simulink model "RangingEstimatorV3Test200CM"  (R2020b)
settings: Solver=FixedStepDiscrete  StartTime=0.0  StopTime=1  FixedStep=0.000001  RelTol=1e-3  EnableMultiTasking=on
settings Model: Creator=拾夕  LastModifiedBy=拾夕
settings OptimizationCC: DefaultUnderspecifiedDataType=single  EnhancedBackFolding=on  PassReuseOutputArgsAs=Individual arguments  ZeroExternalMemoryAtStartup=off  ZeroInternalMemoryAtStartup=off  MaxStackSize=64  OptimizeBlockOrder=speed  DifferentSizesBufferReuse=on  OptimizationCustomize=off  EfficientTunableParamExpr=on
settings DebuggingCC: ParameterTunabilityLossMsg=error
settings HardwareCC: ProdBitPerInt=16  ProdBitPerPointer=16  ProdBitPerSizeT=16  ProdBitPerPtrDiffT=16  ProdLargestAtomicFloat=None  ProdWordSize=8  ProdHWDeviceType=Atmel->AVR
settings SFSimCC: MATLABDynamicMemAlloc=off
settings RTWCC: Description=Embedded Coder  SystemTargetFile=ert.tlc  HardwareBoard=Arduino Uno  TemplateMakefile=ert_default_tmf  GenerateReport=on  RetainRTWFile=on  Toolchain=Arduino AVR  BuildConfiguration=Faster Runs  LaunchReport=on  GenerateWebview=on  GenerateCodeMetricsReport=on
settings CodeAppCC: ForceParamTrailComments=on  IgnoreCustomStorageClasses=off  OperatorAnnotations=on  SimulinkDataObjDesc=on  SFDataObjDesc=on  InsertBlockDesc=on
settings ERTTargetCC: SupportContinuousTime=on  SupportVariableSizeSignals=on  ExtModeStaticAllocSize=250

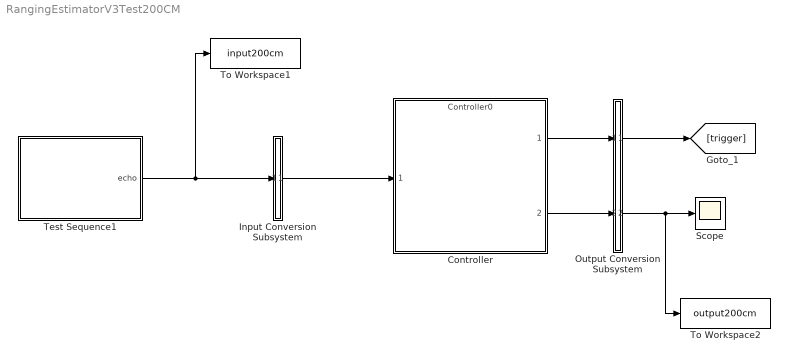
== system RangingEstimatorV3Test200CM ==
  Controller : ModelReference  ModelNameDialog=Controller0  SimulationMode=Normal  ModelReferenceVersion=1.24
  Input Conversion Subsystem : Subsystem  Tag=__SLT_ICS__  Description=|
      | Signal spec.
      | and routing
      settings: AttributesFormatString=%<Description>
  Output Conversion Subsystem : Subsystem  Tag=__SLT_OCS__  Description=|
      | Signal spec.
      | and routing
      settings: AttributesFormatString=%<Description>
  Scope : Scope
  Test Sequence1 : Test Sequence  TreatAsAtomicUnit=on
  To Workspace1 : ToWorkspace  VariableName=input200cm  SaveFormat=Timeseries  SampleTime=-1
  To Workspace2 : ToWorkspace  VariableName=output200cm  SaveFormat=Timeseries  SampleTime=-1
  wires:
  Output Conversion Subsystem/1(Outport_1) -> [trigger]
  Output Conversion Subsystem/2(Outport_2) -> To Workspace2/1, Scope/1
  Input Conversion Subsystem/1(Outport_1) -> Controller/1
  Controller/1 -> Output Conversion Subsystem/1(Inport_1)
  Controller/2 -> Output Conversion Subsystem/2(Inport_2)
  Test Sequence1/1(echo) -> To Workspace1/1, Input Conversion Subsystem/1(Inport_1)

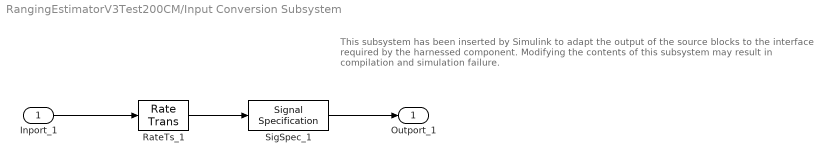
== system RangingEstimatorV3Test200CM/Input Conversion Subsystem ==
  note: This subsystem has been inserted by Simulink to adapt the output of the source blocks to the interface required by the harnessed component.
      |  Modifying the contents of this subsystem may result in compilation and simulation failure.
  Inport_1 : Inport
  RateTs_1 : RateTransition  OutPortSampleTime=1e-06
  SigSpec_1 : SignalSpecification  OutDataTypeStr=single  Dimensions=[1]  SampleTime=1e-06
  Outport_1 : Outport
  wires:
  SigSpec_1/1 -> Outport_1/1
  RateTs_1/1 -> SigSpec_1/1
  Inport_1/1 -> RateTs_1/1

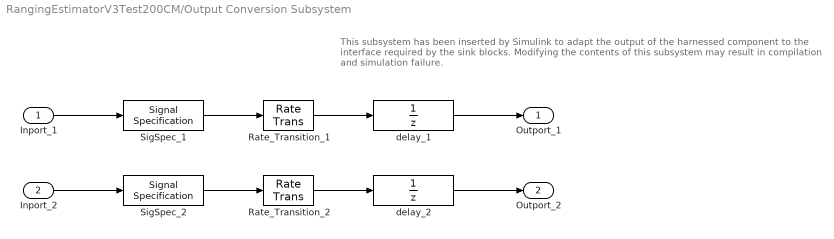
== system RangingEstimatorV3Test200CM/Output Conversion Subsystem ==
  note: This subsystem has been inserted by Simulink to adapt the output of the harnessed component to the interface required by the sink blocks.
      |  Modifying the contents of this subsystem may result in compilation and simulation failure.
  Inport_1 : Inport
  Inport_2 : Inport  Port=2
  Rate_Transition_1 : RateTransition  OutPortSampleTimeOpt=Inherit
  Rate_Transition_2 : RateTransition  OutPortSampleTimeOpt=Inherit
  SigSpec_1 : SignalSpecification  OutDataTypeStr=single  Dimensions=[1]  SampleTime=1e-06
  SigSpec_2 : SignalSpecification  OutDataTypeStr=single  Dimensions=[1]  SampleTime=1e-06
  delay_1 : UnitDelay  SampleTime=-1
  delay_2 : UnitDelay  SampleTime=-1
  Outport_1 : Outport
  Outport_2 : Outport  Port=2
  wires:
  Inport_1/1 -> SigSpec_1/1
  SigSpec_1/1 -> Rate_Transition_1/1
  Rate_Transition_1/1 -> delay_1/1
  delay_1/1 -> Outport_1/1
  Inport_2/1 -> SigSpec_2/1
  SigSpec_2/1 -> Rate_Transition_2/1
  Rate_Transition_2/1 -> delay_2/1
  delay_2/1 -> Outport_2/1

== stateflow chart RangingEstimatorV3Test200CM/Test Sequence1 ==
  settings: stateMachineType=SIMPLIFIED_MACHINE
  state step_1
    echo=1
  state step_2
    echo=0
  (default) -> step_1
  step_1 -> step_2 : [
      | after(58*200,usec)
      | ]
  step_2 -> step_1 : [
      | after(1000*60-58*200,usec)
      | ]
  data: echo output single size=[1]
